simulink model "Schema_inteco"  (R2022b)
settings: Solver=VariableStepAuto  StartTime=0.0  StopTime=60  RelTol=1e-3
undefined symbols (not defined in the file or in its folder): fm, g, Jm, Jphi, kb, kl, L, m, M, R, Ts, w
settings Model: Creator=Bogdana Cazan  LastModifiedBy=Stefi
settings SolverCC: AlgebraicLoopSolver=TrustRegion
settings DataIOCC: ReturnWorkspaceOutputs=off
settings DebuggingCC: UnconnectedInputMsg=warning  UnconnectedOutputMsg=warning  UnconnectedLineMsg=warning  SFMachineParentedDataDiag=warning  ArithmeticOperatorsInVariantConditions=warning
settings ModelReferenceCC: EnableRefExpFcnMdlSchedulingChecks=on
settings SFSimCC: CustomCodeUndefinedFunction=UseInterfaceOnly
settings RTWCC: DLArmComputeVersion=19.05

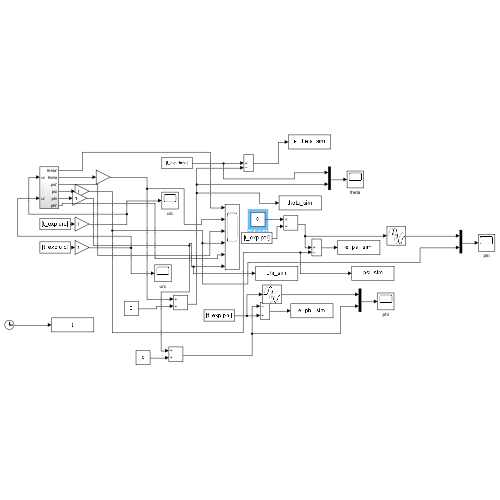
[thumbnail: Simulink's stored preview of the top-level diagram]
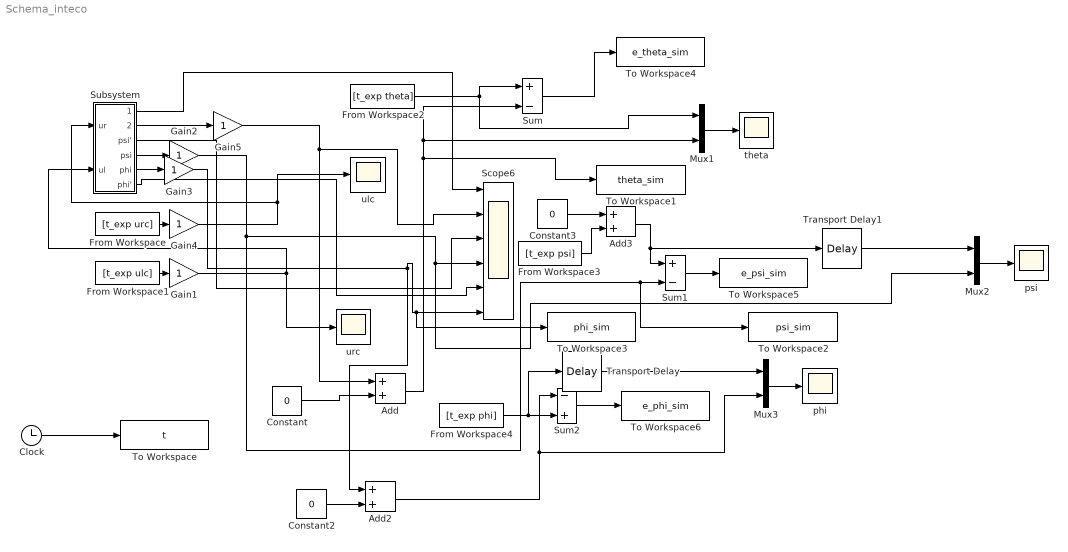
== system Schema_inteco ==
  Add : Sum
  Add2 : Sum
  Add3 : Sum
  Clock : Clock
  Constant : Constant  Value=0
  Constant2 : Constant  Value=0
  Constant3 : Constant  Value=0
  From Workspace : FromWorkspace  VariableName=[t_exp urc]  SampleTime=Ts
  From Workspace1 : FromWorkspace  VariableName=[t_exp ulc]  SampleTime=Ts
  From Workspace2 : FromWorkspace  VariableName=[t_exp theta]  SampleTime=Ts
  From Workspace3 : FromWorkspace  VariableName=[t_exp psi]  SampleTime=Ts
  From Workspace4 : FromWorkspace  VariableName=[t_exp phi]  SampleTime=Ts
  Gain{1..5} (5 alike) : Gain
  Mux1 : Mux  Inputs=2
  Mux2 : Mux  Inputs=2
  Mux3 : Mux  Inputs=2
  Scope6 : Scope  NumInputPorts=6
  Subsystem : Subsystem
  Sum : Sum  Inputs=|+-
  Sum1 : Sum  Inputs=|+-
  Sum2 : Sum  Inputs=-+
  To Workspace : ToWorkspace  VariableName=t  SampleTime=Ts
  To Workspace1 : ToWorkspace  VariableName=theta_sim  SampleTime=Ts
  To Workspace2 : ToWorkspace  VariableName=psi_sim  SampleTime=Ts
  To Workspace3 : ToWorkspace  VariableName=phi_sim  SampleTime=Ts
  To Workspace4 : ToWorkspace  VariableName=e_theta_sim  SampleTime=Ts
  To Workspace5 : ToWorkspace  VariableName=e_psi_sim  SampleTime=Ts
  To Workspace6 : ToWorkspace  VariableName=e_phi_sim  SampleTime=Ts
  Transport Delay : TransportDelay  DelayTime=2.6
  Transport Delay1 : TransportDelay  DelayTime=1.2
  phi : Scope
  psi : Scope
  theta : Scope
  ulc : Scope
  urc : Scope
  wires:
  From Workspace/1 -> Gain4/1
  Subsystem/1(theta') -> Scope6/1
  Subsystem/3(psi') -> Scope6/3
  Subsystem/6(phi') -> Scope6/5
  Clock/1 -> To Workspace/1
  From Workspace2/1 -> Mux1/1, Sum/1
  Sum/1 -> To Workspace4/1
  From Workspace4/1 -> Transport Delay/1, Sum2/2
  Sum2/1 -> To Workspace6/1
  Mux1/1 -> theta/1
  Sum1/1 -> To Workspace5/1
  Mux2/1 -> psi/1
  Mux3/1 -> phi/1
  From Workspace1/1 -> Gain1/1
  Constant/1 -> Add/2
  Add/1 -> To Workspace1/1, Mux1/2, Sum/2
  Constant2/1 -> Add2/2
  Add2/1 -> Mux3/2, Sum2/1
  Gain1/1 -> Subsystem/2(ul), urc/1
  Gain4/1 -> ulc/1, Subsystem/1(ur)
  Subsystem/2(theta) -> Gain5/1
  Subsystem/4(psi) -> Gain2/1
  Subsystem/5(phi) -> Gain3/1
  Gain2/1 -> To Workspace2/1, Sum1/2, Mux2/2, Scope6/4
  Gain3/1 -> To Workspace3/1, Scope6/6, Add2/1
  Gain5/1 -> Add/1, Scope6/2
  Transport Delay/1 -> Mux3/1
  Add3/1 -> Transport Delay1/1, Sum1/1
  From Workspace3/1 -> Add3/2
  Constant3/1 -> Add3/1
  Transport Delay1/1 -> Mux2/1

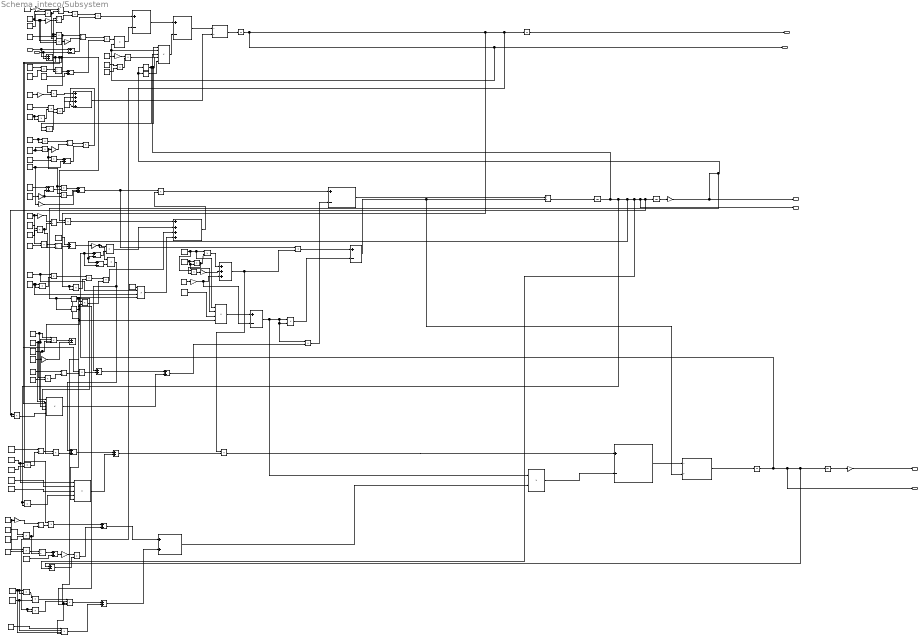
== system Schema_inteco/Subsystem ==
  note: d2
  note: F(psi) primele 2
  note: ftheta
  note: f2
  note: Fpsi
  note: f3 ultimele 2 linii
  note: F3
  note: F2
  note: Theta
  note: Theta' '
  note: Theta'' '
  note: PSI
  note: PSI '
  note: PSI ''
  note: f1
  note: C2
  note: PHI '
  note: d2
  note: UL
  note: UR
  note: C1
  note: PHI
  note: PHI '
  note: PHI ' '
  note: F(fi)
  ur : Inport
  ul : Inport  Port=2
  Add{1,3,11..12,14,17..18,20,22,27..28} (11 alike) : Sum  Inputs=+-
  Add{2,5..6,8,10,13,15,19,21,23..26} (13 alike) : Sum
  Add16 : Sum  Inputs=+++
  Add4 : Sum  Inputs=++++
  Add7 : Sum  Inputs=+++
  Add9 : Sum  Inputs=++++
  Constant{,4,20,27,33,40} (6 alike) : Constant  Value=kl
  Constant{1,14,22,31,39,41,45} (7 alike) : Constant  Value=R
  Constant{2,10,15,19,21,34,42,46} (8 alike) : Constant  Value=m
  Constant{7,11,18,25,30,35,43,52} (8 alike) : Constant  Value=M
  Constant{8..9,12,26,29,36,44,51} (8 alike) : Constant  Value=L
  Constant13 : Constant  Value=w
  Constant16 : Constant  Value=Jm
  Constant17 : Constant  Value=Jphi
  Constant23 : Constant  Value=kb
  Constant24 : Constant  Value=fm
  Constant28 : Constant  Value=g
  Constant3 : Constant  Value=w
  Constant32 : Constant  Value=Jm
  Constant38 : Constant  Value=Jm
  Constant47 : Constant  Value=kb
  Constant48 : Constant  Value=fm
  Constant5 : Constant  Value=kb
  Constant50 : Constant  Value=g
  Constant6 : Constant  Value=fm
  Divide{,1..12,14} (14 alike) : Product  Inputs=*/
  Gain{,1..2,4..6,8..11} (10 alike) : Gain  Gain=2
  Gain12 : Gain  Gain=-1
  Gain13 : Gain  Gain=1/3
  Gain14 : Gain  Gain=-1
  Gain15 : Gain
  Gain16 : Gain
  Gain3 : Gain  Gain=1/2
  Gain7 : Gain  Gain=-1
  Integrator{,1..5} (6 alike) : Integrator
  Product{,1..9,11..32,35..37,39..41,43..47,49..54,56..57,59,61..62} (54 alike) : Product
  Product10 : Product  Inputs=5
  Product{33..34,42,58,60} (5 alike) : Product  Inputs=4
  Product38 : Product  Inputs=5
  Product48 : Product  Inputs=5
  Trigonometric Function : Trigonometry
  Trigonometric Function1 : Trigonometry  Operator=cos
  Trigonometric Function2 : Trigonometry
  Trigonometric Function3 : Trigonometry  Operator=cos
  theta' : Outport  VectorParamsAs1DForOutWhenUnconnected=off
  theta : Outport  Port=2  VectorParamsAs1DForOutWhenUnconnected=off
  psi' : Outport  Port=3  VectorParamsAs1DForOutWhenUnconnected=off
  psi : Outport  Port=4  VectorParamsAs1DForOutWhenUnconnected=off
  phi : Outport  Port=5  VectorParamsAs1DForOutWhenUnconnected=off
  phi' : Outport  Port=6  VectorParamsAs1DForOutWhenUnconnected=off
  wires:
  Constant/1 -> Gain14/1
  Product/1 -> Divide3/2, Divide/2
  Constant1/1 -> Product4/1, Product4/2, Gain/1, Product/1
  Constant2/1 -> Product/2
  Divide/1 -> Product1/1
  Gain/1 -> Divide1/2
  Divide1/1 -> Product1/2
  Product1/1 -> Product2/1
  ur/1 -> Add28/1, Add8/1
  ul/1 -> Add28/2, Add8/2
  Product2/1 -> Add1/1
  Constant3/1 -> Product3/2, Product3/1, Divide1/1
  Product3/1 -> Product11/1, Divide2/1
  Product4/1 -> Gain1/1
  Gain1/1 -> Divide2/2
  Divide2/1 -> Product5/1
  Constant4/1 -> Product6/1
  Constant5/1 -> Product6/2
  Product6/1 -> Divide3/1
  Divide3/1 -> Add2/1
  Constant6/1 -> Add2/2
  Add2/1 -> Product5/2
  Product5/1 -> Product7/1
  Product7/1 -> Add1/2
  Add1/1 -> Add3/1
  Constant7/1 -> Gain2/1
  Gain2/1 -> Product8/1
  Constant8/1 -> Product9/1
  Constant9/1 -> Product9/2
  Product9/1 -> Product8/2
  Product8/1 -> Product10/1
  Product10/1 -> Add3/2
  Trigonometric Function/1 -> Product14/1, Product14/2, Product10/4
  Trigonometric Function1/1 -> Product10/5
  Add3/1 -> Divide4/1
  Constant10/1 -> Gain3/1
  Gain3/1 -> Product11/2
  Product11/1 -> Add4/1
  Constant11/1 -> Product12/1
  Constant12/1 -> Product13/2, Product13/1
  Product13/1 -> Product12/2
  Product14/1 -> Product15/2
  Product12/1 -> Product15/1
  Product15/1 -> Add4/2
  Constant13/1 -> Product16/2, Product16/1
  Constant14/1 -> Product17/1, Product17/2
  Product17/1 -> Product21/1, Product20/1, Product19/1, Gain4/1
  Product16/1 -> Divide5/1
  Gain4/1 -> Divide5/2
  Divide5/1 -> Product18/1
  Constant15/1 -> Product19/2
  Product19/1 -> Add5/1
  Constant16/1 -> Gain6/1, Add5/2
  Add5/1 -> Product18/2
  Product18/1 -> Add4/3
  Constant17/1 -> Add4/4
  Add4/1 -> Divide4/2
  Divide4/1 -> Integrator/1
  Integrator1/1 -> phi/1
  Constant19/1 -> Gain5/1
  Gain5/1 -> Add6/2, Product21/2
  Constant18/1 -> Add6/1
  Add6/1 -> Product20/2
  Product20/1 -> Add7/1
  Product21/1 -> Add7/2
  Gain6/1 -> Add7/3
  Add7/1 -> Product39/1, Product22/1
  Constant20/1 -> Product25/1, Gain7/1
  Constant21/1 -> Product23/1
  Constant22/1 -> Product23/2
  Gain7/1 -> Divide6/1
  Product23/1 -> Divide7/2, Divide6/2
  Divide6/1 -> Product24/2
  Product24/1 -> Add9/1
  Constant23/1 -> Product25/2
  Product25/1 -> Divide7/1
  Divide7/1 -> Add10/2
  Constant24/1 -> Add10/1
  Gain8/1 -> Product47/1, Product26/1
  Constant26/1 -> Product33/3, Product27/2, Product27/1
  Constant25/1 -> Product33/2, Product28/1
  Product27/1 -> Product28/2
  Product28/1 -> Product29/1
  Product30/1 -> Product29/2
  Product29/1 -> Product31/1
  Product32/1 -> Product31/2
  Product31/1 -> Add9/3
  Constant28/1 -> Product33/1
  Product33/1 -> Add9/4
  Add9/1 -> Product22/2
  Product22/1 -> Add11/1
  Constant30/1 -> Product38/1, Product34/1
  Constant31/1 -> Product36/1, Product38/2, Product34/2
  Constant29/1 -> Product38/3, Product34/3
  Product34/1 -> Add12/1
  Constant32/1 -> Gain9/1
  Gain9/1 -> Add12/2
  Constant33/1 -> Divide8/1
  Constant34/1 -> Product36/2
  Product36/1 -> Divide8/2
  Divide8/1 -> Product37/2
  Product37/1 -> Add13/2
  Integrator5/1 -> Gain15/1
  Add14/1 -> Product26/2
  Product26/1 -> Add9/2
  Add13/1 -> Add15/1
  Product38/1 -> Add15/2
  Add15/1 -> Product35/2
  Product35/1 -> Add11/2
  Add11/1 -> Divide9/1
  Constant36/1 -> Product42/2, Product41/2, Product41/1
  Constant35/1 -> Product54/1, Product42/1, Product40/1
  Product41/1 -> Product54/2, Product40/2
  Product40/1 -> Add16/1
  Product54/1 -> Gain13/1
  Constant38/1 -> Gain10/1
  Gain10/1 -> Add18/2, Add16/3
  Product39/1 -> Add17/1
  Constant39/1 -> Product42/3
  Product42/1 -> Add18/1
  Product43/1 -> Add17/2
  Divide9/1 -> Integrator2/1
  Add16/1 -> Product39/2, Product44/1
  Constant41/1 -> Product48/1, Product45/1
  Constant42/1 -> Product45/2
  Constant40/1 -> Divide10/1
  Product45/1 -> Divide10/2
  Divide10/1 -> Product46/1
  Product46/1 -> Add19/2
  Add20/1 -> Product47/2
  Product47/1 -> Add13/1, Add19/1
  Add19/1 -> Add21/1
  Constant43/1 -> Product48/2
  Constant44/1 -> Product48/3
  Product48/1 -> Add21/2
  Add21/1 -> Product44/2
  Product44/1 -> Add22/1
  Add10/1 -> Gain8/1
  Constant52/1 -> Product60/2, Product56/2
  Constant51/1 -> Product60/3, Product57/2, Product57/1
  Product57/1 -> Product56/1
  Product56/1 -> Product58/1
  Product59/1 -> Product58/2
  Trigonometric Function3/1 -> Product58/4, Product32/2, Product34/4, Product42/4
  Product58/1 -> Add25/1
  Constant50/1 -> Product60/1
  Product60/1 -> Add25/2
  Add25/1 -> Add24/2
  Add24/1 -> Product49/2
  Product49/1 -> Add22/2
  Add22/1 -> Divide14/1
  Add17/1 -> Divide14/2, Divide9/2
  Divide14/1 -> Integrator4/1
  Product61/1 -> Product38/5
  Product62/1 -> Product48/4
  Trigonometric Function2/1 -> Product48/5, Product38/4, Product32/1, Product33/4, Product60/4, Product58/3
  Constant45/1 -> Product50/1
  Constant46/1 -> Product50/2
  Constant27/1 -> Product52/1, Gain12/1
  Product50/1 -> Divide12/2, Divide11/2
  Divide11/1 -> Product51/2
  Product51/1 -> Add23/1
  Constant47/1 -> Product52/2
  Product52/1 -> Divide12/1
  Divide12/1 -> Add26/1
  Constant48/1 -> Add26/2
  Add26/1 -> Gain11/1
  Gain11/1 -> Product53/1
  Add27/1 -> Product53/2
  Product53/1 -> Add23/2
  Add23/1 -> Add24/1
  Gain12/1 -> Divide11/1
  Integrator4/1 -> Add20/2, Add14/1, theta'/1, Add27/1, Integrator5/1
  Gain13/1 -> Add16/2
  Integrator2/1 -> Product62/2, Product62/1, Add27/2, Product61/2, Product61/1, Integrator3/1, psi'/1, Add20/1, Add14/2, Product10/3
  Integrator/1 -> Product7/2, Product10/2, phi'/1, Product30/1, Product30/2, Product59/2, Product59/1, Integrator1/1
  Gain14/1 -> Divide/1
  Add18/1 -> Product49/1, Product35/1, Product43/2, Product43/1
  Integrator3/1 -> Gain16/1
  Gain15/1 -> theta/1
  Gain16/1 -> Trigonometric Function3/1, Trigonometric Function2/1, Trigonometric Function1/1, Trigonometric Function/1, psi/1
  Add8/1 -> Product37/1, Product46/2, Product51/1, Product24/1
  Add28/1 -> Product2/2
